simulink model "DCPositionaCS"  (R2020a)
settings: Solver=VariableStepAuto  StartTime=0.0  StopTime=10.0  RelTol=1e-3
settings Model: Creator=Pranshu  LastModifiedBy=Pranshu

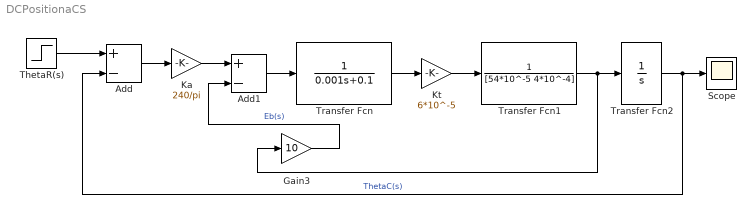
== system DCPositionaCS ==
  Add : Sum  Inputs=+|-
  Add1 : Sum  Inputs=+|-
  Gain3 : Gain  Gain=10
  Ka : Gain  Gain=240/pi
  Kt : Gain  Gain=6*10^-5
  Scope : Scope
  ThetaR(s) : Step  Time=0  SampleTime=0
  Transfer Fcn : TransferFcn  Denominator=[0.001 0.1]
  Transfer Fcn1 : TransferFcn  Denominator=[54*10^-5 4*10^-4]
  Transfer Fcn2 : TransferFcn  Denominator=[1 0]
  wires:
  ThetaR(s)/1 -> Add/1
  Kt/1 -> Transfer Fcn1/1
  Transfer Fcn/1 -> Kt/1
  Add/1 -> Ka/1
  Transfer Fcn2/1 -> Add/2, Scope/1  "ThetaC(s)"
  Add1/1 -> Transfer Fcn/1
  Gain3/1 -> Add1/2  "Eb(s)"
  Transfer Fcn1/1 -> Gain3/1, Transfer Fcn2/1
  Ka/1 -> Add1/1
